simulink model "motorTest"  (R2016a)
settings: Solver=FixedStepDiscrete  StartTime=0.0  StopTime=Inf  RelTol=1e-3
libraries: simulink x2
settings Model: SimulationMode=external  ExtModeTrigDuration=2  Creator=shohei  LastModifiedBy=shohei
settings OptimizationCC: OptimizeModelRefInitCode=on  LifeSpan=1  MaxStackSize=64
settings HardwareCC: ProdBitPerInt=16  ProdBitPerPointer=16  ProdLargestAtomicFloat=None  ProdWordSize=8  ProdHWDeviceType=Atmel->AVR
settings RTWCC: SystemTargetFile=ert.tlc  HardwareBoard=Arduino Mega 2560  TemplateMakefile=ert_default_tmf  GenerateReport=on  Toolchain=Arduino AVR v1.6.1  BuildConfiguration=Faster Runs  IncludeHyperlinkInReport=on  LaunchReport=on  GenerateTraceInfo=on  GenerateTraceReport=on  GenerateTraceReportSl=on  GenerateTraceReportSf=on  GenerateTraceReportEml=on
settings CodeAppCC: ForceParamTrailComments=on  IgnoreCustomStorageClasses=off  OperatorAnnotations=on  SimulinkDataObjDesc=on  SFDataObjDesc=on  MATLABFcnDesc=on  InsertBlockDesc=on  MATLABSourceComments=on
settings ERTTargetCC: SupportContinuousTime=on  SupportVariableSizeSignals=on

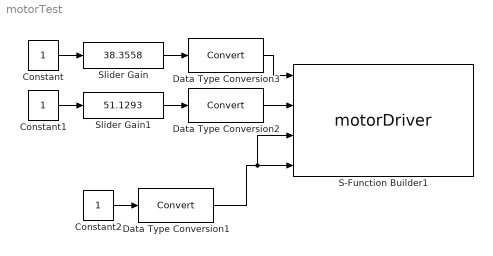
== system motorTest ==
  Constant : Constant
  Constant1 : Constant
  Constant2 : Constant
  Data Type Conversion1 : DataTypeConversion
  Data Type Conversion2 : DataTypeConversion
  Data Type Conversion3 : DataTypeConversion
  S-Function Builder1 : S-Function  InitFcn=try, set_param(gcb,'FunctionName','motorDriver'), end  FunctionName=motorDriver  SFunctionModules=motorDriver_wrapper  SFunctionDeploymentMode=off  EnableBusSupport=off  mask(S-Function Builder){}
      mask help: Simulink:masks:SFunctionBuilder_MD
      mask init:
      | val = [[.9  0.75 0.75 1 1 .9 .9 1]',[1 1 0.75 0.75 .9 .9 1 .9]'];try , sys = get_param(gcb,'SfunBuilderFcnName');if isempty(sys), sys = get_param(gcb,'FunctionName'); end,catch, sys = get_param(gcb,'FunctionName'); end
      settings: CopyFcn=set_param(gcbh,'LinkStatus','none')  PreSaveFcn=try, set_param(gcb,'FunctionName','motorDriver'), end  OpenFcn=sfunctionwizard(gcbh)
      mask Display: plot(val(:,1),val(:,2)),disp(sys), port_label('input',1,'speed1'), port_label('input',2,'speed2'), port_label('input',3,'direction1'), port_label('input',4,'direction2')
  Slider Gain : simulink/Math Operations/Slider Gain  low=0  gain=38.3558  high=255
  Slider Gain1 : simulink/Math Operations/Slider Gain  low=0  gain=51.1293  high=255
  wires:
  Constant2/1 -> Data Type Conversion1/1
  Data Type Conversion1/1 -> S-Function Builder1/4, S-Function Builder1/3
  Data Type Conversion2/1 -> S-Function Builder1/2
  Slider Gain1/1 -> Data Type Conversion2/1
  Data Type Conversion3/1 -> S-Function Builder1/1
  Slider Gain/1 -> Data Type Conversion3/1
  Constant/1 -> Slider Gain/1
  Constant1/1 -> Slider Gain1/1
